simulink model "c6_goto_target"  (R2021b)
settings: Solver=FixedStepDiscrete  StartTime=0.0  StopTime=Inf  FixedStep=sampleTime  RelTol=1e-3  EnableMultiTasking=on
PreLoadFcn:
  | %load emptyMap
InitFcn:
  | sampleTime = 0.05;
  | nMedianSize=3;
  | %load boundaryMap
  | 
  | % Robot parameters
  | wheelRadius = 0.0303;
  | robotRadius = 0.06;   %小车在仿真中显示的圆形的半径大小
  | Trackwidth = 0.0847;  %定义向量场直方图算法中小车的宽度
  | 
  | % Lidar parameters
  | sensorOffset = [0,0];
  | scanAngles = linspace(-pi/3,pi/3,20)';%y = linspace(x1,x2,n) 生成 n 个点。这些点的间距为 (x2-x1)/(n-1)。
  | maxRange = 0.4;
  | 
  | %%%%%%
  | ks=1;
  | 
  | 
  | 
  | 
  | 
  | A=0.5;
  | C=1.5;
  | B=(A+C)/2;
  | 
  | wp1=[A,A; B,A;  C,A; C,B;C,C; B,C; A,C;A,B];
  | bainjie2=[-0.5,-0.5;2.5,-0.5;-0.5,2.5;2.5,2.5;]
  | WAY_P=[wp1;wp1;wp1;wp1];
  | Target=[wp1;bainjie2];
  | 
  | %%%%%%%%%%%%%%%%%%%%%%%%%%%%%%%%%%%%%%%
  | Target_robot_4=[A  A]
  | Target_robot_5=[B  A]
  | Target_robot_6=[C  A]
  | 
  | Target_robot_1=[C  C]
  | Target_robot_2=[B  C]
  | Target_robot_3=[A  C]
  | 
  | 
  | %%%%%%%%%%%%%%%%%%%%%%%%%%%%%%%%%%%%
  | 
  | 
  | init_pose_1=[A    A  pi/2]';
  | init_pose_2=[B    A  pi/2]';
  | init_pose_3=[C    A  pi/2]';
  | init_pose_4=[C    C  -pi/2]';
  | init_pose_5=[B    C  -pi/2]';
  | init_pose_6=[A    C  -pi/2]';
  | 
  | 
  | 
  | 
  | %{
  | %初始位置 交叉
  | 
  | init_pose_1=[C    C    0]';
  | init_pose_2=[B    C    0]';
  | init_pose_3=[A    C  0]';
  | init_pose_4=[A    A  0]';
  | ... (+26 lines)
undefined symbols (not defined in the file or in its folder): Angular, DiscIntNeverNeededParam, Linear
libraries: robotlib x27, dspstat3 x18, robotalgslib x12
(part 2 of 3)

== system c6_goto_target/controller1/Subsystem2/Compute Velocity and Heading for Path following ==
  note: Check If Close To Goal
  CurrentPose : Inport
  Waypoints : Inport  Port=2
  " Extract Goal" : MATLAB Function  TreatAsAtomicUnit=on
  Dot Product : DotProduct  InputSameDT=on  OutDataTypeStr=Inherit: Inherit via internal rule
  GoalRadius : Constant  Value=0.1
  Pure Pursuit : robotalgslib/Pure Pursuit  DesiredLinearVelocity=desired_v  MaxAngularVelocity=desired_w  LookaheadDistance=desired_lookahead  TargetDirPort=on  SimulateUsing=Code generation
  Relational Operator : RelationalOperator  Operator=<=  OutDataTypeStr=boolean  RndMeth=Simplest
  Selector : Selector  InputPortWidth=3  IndexOptions=Index vector (dialog)  Indices=[1 2]  OutputSizes=1
  Sqrt : Sqrt  SaturateOnIntegerOverflow=on
  Subtract : Sum  Inputs=+-
  TargetDir : Outport  VectorParamsAs1DForOutWhenUnconnected=off
  V : Outport  Port=2  VectorParamsAs1DForOutWhenUnconnected=off
  W : Outport  Port=3  VectorParamsAs1DForOutWhenUnconnected=off
  CloseToGoal : Outport  Port=4  VectorParamsAs1DForOutWhenUnconnected=off
  wires:
  Pure Pursuit/3 -> TargetDir/1
  Pure Pursuit/2 -> W/1
  Pure Pursuit/1 -> V/1
  " Extract Goal"/1(Goal) -> Subtract/2
  Waypoints/1 -> " Extract Goal"/1(Waypoints), Pure Pursuit/2
  CurrentPose/1 -> Selector/1, Pure Pursuit/1
  Relational Operator/1 -> CloseToGoal/1
  GoalRadius/1 -> Relational Operator/2
  Selector/1 -> Subtract/1
  Dot Product/1 -> Sqrt/1
  Sqrt/1 -> Relational Operator/1
  Subtract/1 -> Dot Product/1, Dot Product/2

== system c6_goto_target/controller1/Subsystem2/More Info ==

== system c6_goto_target/controller1/Subsystem2/Outputs ==
  dV : Inport
  dW : Inport  Port=2
  V : Inport  Port=3
  W : Inport  Port=4
  CloseToGoal : Inport  Port=5
  Add : Sum
  Add1 : Sum
  Logical Operator : Logic  Operator=NOT  AllPortsSameDT=off  OutDataTypeStr=boolean
  Product : Product
  Product1 : Product
  v : Outport
  w : Outport  Port=2
  wires:
  V/1 -> Add/2
  W/1 -> Add1/2
  dV/1 -> Add/1
  dW/1 -> Add1/1
  CloseToGoal/1 -> Logical Operator/1
  Add/1 -> Product/1
  Add1/1 -> Product1/1
  Product1/1 -> w/1
  Product/1 -> v/1
  Logical Operator/1 -> Product1/2, Product/2

== system c6_goto_target/controller1/Subsystem3/Adjust Velocities to Avoid Obstacles ==
  note: Based on proposed steering direction, evaluate feasible velocities (linear and angular).
      | 				Switch to recovery behavior if no feasible steering direction.
  Ranges : Inport
  Angles : Inport  Port=2
  TargetDir : Inport  Port=3
  V : Inport  Port=4
  W : Inport  Port=5
  If : If  IfExpression=u1 == 1
  Merge : Merge
  Merge1 : Merge
  Path Following : Subsystem  TreatAsAtomicUnit=on
  Recovery : Subsystem  TreatAsAtomicUnit=on
  Relational Operator : RelationalOperator  Operator=isNaN  OutDataTypeStr=boolean  RndMeth=Simplest
  Vector Field Histogram : robotalgslib/Vector Field Histogram  NumAngularSectors=180  DistanceLimits=[ 0.05, 3 ]  HistogramThresholds=[ 3, 8 ]  RobotRadius=0.2  SafetyDistance=0.2  MinTurningRadius=0.2  SimulateUsing=Code generation  TargetDirectionWeight=5  CurrentDirectionWeight=2  PreviousDirectionWeight=2
      settings: SourceProductBaseCode=NV,RO
  dV : Outport  VectorParamsAs1DForOutWhenUnconnected=off
  dW : Outport  Port=2  VectorParamsAs1DForOutWhenUnconnected=off
  wires:
  Merge1/1 -> dW/1
  V/1 -> Recovery/1(LinearVelocity)
  Vector Field Histogram/1 -> Relational Operator/1, Path Following/1(SteeringDirection)
  W/1 -> Recovery/2(AngularVelocity), Path Following/2(AngularVelocity)
  Relational Operator/1 -> If/1
  Angles/1 -> Vector Field Histogram/2
  Merge/1 -> dV/1
  TargetDir/1 -> Vector Field Histogram/3
  Ranges/1 -> Vector Field Histogram/1
  If/1 -> Recovery/Action
  If/2 -> Path Following/Action
  Recovery/2(dW) -> Merge1/1
  Path Following/2(dW) -> Merge1/2
  Recovery/1(dV) -> Merge/1
  Path Following/1(dV) -> Merge/2

== system c6_goto_target/controller1/Subsystem3/Compute Velocity and Heading for Path following ==
  note: Check If Close To Goal
  CurrentPose : Inport
  Waypoints : Inport  Port=2
  " Extract Goal" : MATLAB Function  TreatAsAtomicUnit=on
  Dot Product : DotProduct  InputSameDT=on  OutDataTypeStr=Inherit: Inherit via internal rule
  GoalRadius : Constant  Value=0.1
  Pure Pursuit : robotalgslib/Pure Pursuit  DesiredLinearVelocity=desired_v  MaxAngularVelocity=desired_w  LookaheadDistance=desired_lookahead  TargetDirPort=on  SimulateUsing=Code generation
  Relational Operator : RelationalOperator  Operator=<=  OutDataTypeStr=boolean  RndMeth=Simplest
  Selector : Selector  InputPortWidth=3  IndexOptions=Index vector (dialog)  Indices=[1 2]  OutputSizes=1
  Sqrt : Sqrt  SaturateOnIntegerOverflow=on
  Subtract : Sum  Inputs=+-
  TargetDir : Outport  VectorParamsAs1DForOutWhenUnconnected=off
  V : Outport  Port=2  VectorParamsAs1DForOutWhenUnconnected=off
  W : Outport  Port=3  VectorParamsAs1DForOutWhenUnconnected=off
  CloseToGoal : Outport  Port=4  VectorParamsAs1DForOutWhenUnconnected=off
  wires:
  Pure Pursuit/3 -> TargetDir/1
  Pure Pursuit/2 -> W/1
  Pure Pursuit/1 -> V/1
  " Extract Goal"/1(Goal) -> Subtract/2
  Waypoints/1 -> " Extract Goal"/1(Waypoints), Pure Pursuit/2
  CurrentPose/1 -> Selector/1, Pure Pursuit/1
  Relational Operator/1 -> CloseToGoal/1
  GoalRadius/1 -> Relational Operator/2
  Selector/1 -> Subtract/1
  Dot Product/1 -> Sqrt/1
  Sqrt/1 -> Relational Operator/1
  Subtract/1 -> Dot Product/1, Dot Product/2

== system c6_goto_target/controller1/Subsystem3/More Info ==

== system c6_goto_target/controller1/Subsystem3/Outputs ==
  dV : Inport
  dW : Inport  Port=2
  V : Inport  Port=3
  W : Inport  Port=4
  CloseToGoal : Inport  Port=5
  Add : Sum
  Add1 : Sum
  Logical Operator : Logic  Operator=NOT  AllPortsSameDT=off  OutDataTypeStr=boolean
  Product : Product
  Product1 : Product
  v : Outport
  w : Outport  Port=2
  wires:
  V/1 -> Add/2
  W/1 -> Add1/2
  dV/1 -> Add/1
  dW/1 -> Add1/1
  CloseToGoal/1 -> Logical Operator/1
  Add/1 -> Product/1
  Add1/1 -> Product1/1
  Product1/1 -> w/1
  Product/1 -> v/1
  Logical Operator/1 -> Product1/2, Product/2

== system c6_goto_target/controller1/Subsystem4/Adjust Velocities to Avoid Obstacles ==
  note: Based on proposed steering direction, evaluate feasible velocities (linear and angular).
      | 				Switch to recovery behavior if no feasible steering direction.
  Ranges : Inport
  Angles : Inport  Port=2
  TargetDir : Inport  Port=3
  V : Inport  Port=4
  W : Inport  Port=5
  If : If  IfExpression=u1 == 1
  Merge : Merge
  Merge1 : Merge
  Path Following : Subsystem  TreatAsAtomicUnit=on
  Recovery : Subsystem  TreatAsAtomicUnit=on
  Relational Operator : RelationalOperator  Operator=isNaN  OutDataTypeStr=boolean  RndMeth=Simplest
  Vector Field Histogram : robotalgslib/Vector Field Histogram  NumAngularSectors=180  DistanceLimits=[ 0.05, 3 ]  HistogramThresholds=[ 3, 8 ]  RobotRadius=0.2  SafetyDistance=0.2  MinTurningRadius=0.2  SimulateUsing=Code generation  TargetDirectionWeight=5  CurrentDirectionWeight=2  PreviousDirectionWeight=2
      settings: SourceProductBaseCode=NV,RO
  dV : Outport  VectorParamsAs1DForOutWhenUnconnected=off
  dW : Outport  Port=2  VectorParamsAs1DForOutWhenUnconnected=off
  wires:
  Merge1/1 -> dW/1
  V/1 -> Recovery/1(LinearVelocity)
  Vector Field Histogram/1 -> Relational Operator/1, Path Following/1(SteeringDirection)
  W/1 -> Recovery/2(AngularVelocity), Path Following/2(AngularVelocity)
  Relational Operator/1 -> If/1
  Angles/1 -> Vector Field Histogram/2
  Merge/1 -> dV/1
  TargetDir/1 -> Vector Field Histogram/3
  Ranges/1 -> Vector Field Histogram/1
  If/1 -> Recovery/Action
  If/2 -> Path Following/Action
  Recovery/2(dW) -> Merge1/1
  Path Following/2(dW) -> Merge1/2
  Recovery/1(dV) -> Merge/1
  Path Following/1(dV) -> Merge/2

== system c6_goto_target/controller1/Subsystem4/Compute Velocity and Heading for Path following ==
  note: Check If Close To Goal
  CurrentPose : Inport
  Waypoints : Inport  Port=2
  " Extract Goal" : MATLAB Function  TreatAsAtomicUnit=on
  Dot Product : DotProduct  InputSameDT=on  OutDataTypeStr=Inherit: Inherit via internal rule
  GoalRadius : Constant  Value=0.1
  Pure Pursuit : robotalgslib/Pure Pursuit  DesiredLinearVelocity=desired_v  MaxAngularVelocity=desired_w  LookaheadDistance=desired_lookahead  TargetDirPort=on  SimulateUsing=Code generation
  Relational Operator : RelationalOperator  Operator=<=  OutDataTypeStr=boolean  RndMeth=Simplest
  Selector : Selector  InputPortWidth=3  IndexOptions=Index vector (dialog)  Indices=[1 2]  OutputSizes=1
  Sqrt : Sqrt  SaturateOnIntegerOverflow=on
  Subtract : Sum  Inputs=+-
  TargetDir : Outport  VectorParamsAs1DForOutWhenUnconnected=off
  V : Outport  Port=2  VectorParamsAs1DForOutWhenUnconnected=off
  W : Outport  Port=3  VectorParamsAs1DForOutWhenUnconnected=off
  CloseToGoal : Outport  Port=4  VectorParamsAs1DForOutWhenUnconnected=off
  wires:
  Pure Pursuit/3 -> TargetDir/1
  Pure Pursuit/2 -> W/1
  Pure Pursuit/1 -> V/1
  " Extract Goal"/1(Goal) -> Subtract/2
  Waypoints/1 -> " Extract Goal"/1(Waypoints), Pure Pursuit/2
  CurrentPose/1 -> Selector/1, Pure Pursuit/1
  Relational Operator/1 -> CloseToGoal/1
  GoalRadius/1 -> Relational Operator/2
  Selector/1 -> Subtract/1
  Dot Product/1 -> Sqrt/1
  Sqrt/1 -> Relational Operator/1
  Subtract/1 -> Dot Product/1, Dot Product/2

== system c6_goto_target/controller1/Subsystem4/More Info ==

== system c6_goto_target/controller1/Subsystem4/Outputs ==
  dV : Inport
  dW : Inport  Port=2
  V : Inport  Port=3
  W : Inport  Port=4
  CloseToGoal : Inport  Port=5
  Add : Sum
  Add1 : Sum
  Logical Operator : Logic  Operator=NOT  AllPortsSameDT=off  OutDataTypeStr=boolean
  Product : Product
  Product1 : Product
  v : Outport
  w : Outport  Port=2
  wires:
  V/1 -> Add/2
  W/1 -> Add1/2
  dV/1 -> Add/1
  dW/1 -> Add1/1
  CloseToGoal/1 -> Logical Operator/1
  Add/1 -> Product/1
  Add1/1 -> Product1/1
  Product1/1 -> w/1
  Product/1 -> v/1
  Logical Operator/1 -> Product1/2, Product/2

== system c6_goto_target/controller1/Subsystem5/Adjust Velocities to Avoid Obstacles ==
  note: Based on proposed steering direction, evaluate feasible velocities (linear and angular).
      | 				Switch to recovery behavior if no feasible steering direction.
  Ranges : Inport
  Angles : Inport  Port=2
  TargetDir : Inport  Port=3
  V : Inport  Port=4
  W : Inport  Port=5
  If : If  IfExpression=u1 == 1
  Merge : Merge
  Merge1 : Merge
  Path Following : Subsystem  TreatAsAtomicUnit=on
  Recovery : Subsystem  TreatAsAtomicUnit=on
  Relational Operator : RelationalOperator  Operator=isNaN  OutDataTypeStr=boolean  RndMeth=Simplest
  Vector Field Histogram : robotalgslib/Vector Field Histogram  NumAngularSectors=180  DistanceLimits=[ 0.05, 3 ]  HistogramThresholds=[ 3, 8 ]  RobotRadius=0.2  SafetyDistance=0.2  MinTurningRadius=0.2  SimulateUsing=Code generation  TargetDirectionWeight=5  CurrentDirectionWeight=2  PreviousDirectionWeight=2
      settings: SourceProductBaseCode=NV,RO
  dV : Outport  VectorParamsAs1DForOutWhenUnconnected=off
  dW : Outport  Port=2  VectorParamsAs1DForOutWhenUnconnected=off
  wires:
  Merge1/1 -> dW/1
  V/1 -> Recovery/1(LinearVelocity)
  Vector Field Histogram/1 -> Relational Operator/1, Path Following/1(SteeringDirection)
  W/1 -> Recovery/2(AngularVelocity), Path Following/2(AngularVelocity)
  Relational Operator/1 -> If/1
  Angles/1 -> Vector Field Histogram/2
  Merge/1 -> dV/1
  TargetDir/1 -> Vector Field Histogram/3
  Ranges/1 -> Vector Field Histogram/1
  If/1 -> Recovery/Action
  If/2 -> Path Following/Action
  Recovery/2(dW) -> Merge1/1
  Path Following/2(dW) -> Merge1/2
  Recovery/1(dV) -> Merge/1
  Path Following/1(dV) -> Merge/2

== system c6_goto_target/controller1/Subsystem5/Compute Velocity and Heading for Path following ==
  note: Check If Close To Goal
  CurrentPose : Inport
  Waypoints : Inport  Port=2
  " Extract Goal" : MATLAB Function  TreatAsAtomicUnit=on
  Dot Product : DotProduct  InputSameDT=on  OutDataTypeStr=Inherit: Inherit via internal rule
  GoalRadius : Constant  Value=0.1
  Pure Pursuit : robotalgslib/Pure Pursuit  DesiredLinearVelocity=desired_v  MaxAngularVelocity=desired_w  LookaheadDistance=desired_lookahead  TargetDirPort=on  SimulateUsing=Code generation
  Relational Operator : RelationalOperator  Operator=<=  OutDataTypeStr=boolean  RndMeth=Simplest
  Selector : Selector  InputPortWidth=3  IndexOptions=Index vector (dialog)  Indices=[1 2]  OutputSizes=1
  Sqrt : Sqrt  SaturateOnIntegerOverflow=on
  Subtract : Sum  Inputs=+-
  TargetDir : Outport  VectorParamsAs1DForOutWhenUnconnected=off
  V : Outport  Port=2  VectorParamsAs1DForOutWhenUnconnected=off
  W : Outport  Port=3  VectorParamsAs1DForOutWhenUnconnected=off
  CloseToGoal : Outport  Port=4  VectorParamsAs1DForOutWhenUnconnected=off
  wires:
  Pure Pursuit/3 -> TargetDir/1
  Pure Pursuit/2 -> W/1
  Pure Pursuit/1 -> V/1
  " Extract Goal"/1(Goal) -> Subtract/2
  Waypoints/1 -> " Extract Goal"/1(Waypoints), Pure Pursuit/2
  CurrentPose/1 -> Selector/1, Pure Pursuit/1
  Relational Operator/1 -> CloseToGoal/1
  GoalRadius/1 -> Relational Operator/2
  Selector/1 -> Subtract/1
  Dot Product/1 -> Sqrt/1
  Sqrt/1 -> Relational Operator/1
  Subtract/1 -> Dot Product/1, Dot Product/2

== system c6_goto_target/controller1/Subsystem5/More Info ==

== system c6_goto_target/controller1/Subsystem5/Outputs ==
  dV : Inport
  dW : Inport  Port=2
  V : Inport  Port=3
  W : Inport  Port=4
  CloseToGoal : Inport  Port=5
  Add : Sum
  Add1 : Sum
  Logical Operator : Logic  Operator=NOT  AllPortsSameDT=off  OutDataTypeStr=boolean
  Product : Product
  Product1 : Product
  v : Outport
  w : Outport  Port=2
  wires:
  V/1 -> Add/2
  W/1 -> Add1/2
  dV/1 -> Add/1
  dW/1 -> Add1/1
  CloseToGoal/1 -> Logical Operator/1
  Add/1 -> Product/1
  Add1/1 -> Product1/1
  Product1/1 -> w/1
  Product/1 -> v/1
  Logical Operator/1 -> Product1/2, Product/2

== system c6_goto_target/controller1/Subsystem6/Adjust Velocities to Avoid Obstacles ==
  note: Based on proposed steering direction, evaluate feasible velocities (linear and angular).
      | 				Switch to recovery behavior if no feasible steering direction.
  Ranges : Inport
  Angles : Inport  Port=2
  TargetDir : Inport  Port=3
  V : Inport  Port=4
  W : Inport  Port=5
  If : If  IfExpression=u1 == 1
  Merge : Merge
  Merge1 : Merge
  Path Following : Subsystem  TreatAsAtomicUnit=on
  Recovery : Subsystem  TreatAsAtomicUnit=on
  Relational Operator : RelationalOperator  Operator=isNaN  OutDataTypeStr=boolean  RndMeth=Simplest
  Vector Field Histogram : robotalgslib/Vector Field Histogram  NumAngularSectors=180  DistanceLimits=[ 0.05, 3 ]  HistogramThresholds=[ 3, 8 ]  RobotRadius=0.2  SafetyDistance=0.2  MinTurningRadius=0.2  SimulateUsing=Code generation  TargetDirectionWeight=5  CurrentDirectionWeight=2  PreviousDirectionWeight=2
      settings: SourceProductBaseCode=NV,RO
  dV : Outport  VectorParamsAs1DForOutWhenUnconnected=off
  dW : Outport  Port=2  VectorParamsAs1DForOutWhenUnconnected=off
  wires:
  Merge1/1 -> dW/1
  V/1 -> Recovery/1(LinearVelocity)
  Vector Field Histogram/1 -> Relational Operator/1, Path Following/1(SteeringDirection)
  W/1 -> Recovery/2(AngularVelocity), Path Following/2(AngularVelocity)
  Relational Operator/1 -> If/1
  Angles/1 -> Vector Field Histogram/2
  Merge/1 -> dV/1
  TargetDir/1 -> Vector Field Histogram/3
  Ranges/1 -> Vector Field Histogram/1
  If/1 -> Recovery/Action
  If/2 -> Path Following/Action
  Recovery/2(dW) -> Merge1/1
  Path Following/2(dW) -> Merge1/2
  Recovery/1(dV) -> Merge/1
  Path Following/1(dV) -> Merge/2

== system c6_goto_target/controller1/Subsystem6/Compute Velocity and Heading for Path following ==
  note: Check If Close To Goal
  CurrentPose : Inport
  Waypoints : Inport  Port=2
  " Extract Goal" : MATLAB Function  TreatAsAtomicUnit=on
  Dot Product : DotProduct  InputSameDT=on  OutDataTypeStr=Inherit: Inherit via internal rule
  GoalRadius : Constant  Value=0.1
  Pure Pursuit : robotalgslib/Pure Pursuit  DesiredLinearVelocity=desired_v  MaxAngularVelocity=desired_w  LookaheadDistance=desired_lookahead  TargetDirPort=on  SimulateUsing=Code generation
  Relational Operator : RelationalOperator  Operator=<=  OutDataTypeStr=boolean  RndMeth=Simplest
  Selector : Selector  InputPortWidth=3  IndexOptions=Index vector (dialog)  Indices=[1 2]  OutputSizes=1
  Sqrt : Sqrt  SaturateOnIntegerOverflow=on
  Subtract : Sum  Inputs=+-
  TargetDir : Outport  VectorParamsAs1DForOutWhenUnconnected=off
  V : Outport  Port=2  VectorParamsAs1DForOutWhenUnconnected=off
  W : Outport  Port=3  VectorParamsAs1DForOutWhenUnconnected=off
  CloseToGoal : Outport  Port=4  VectorParamsAs1DForOutWhenUnconnected=off
  wires:
  Pure Pursuit/3 -> TargetDir/1
  Pure Pursuit/2 -> W/1
  Pure Pursuit/1 -> V/1
  " Extract Goal"/1(Goal) -> Subtract/2
  Waypoints/1 -> " Extract Goal"/1(Waypoints), Pure Pursuit/2
  CurrentPose/1 -> Selector/1, Pure Pursuit/1
  Relational Operator/1 -> CloseToGoal/1
  GoalRadius/1 -> Relational Operator/2
  Selector/1 -> Subtract/1
  Dot Product/1 -> Sqrt/1
  Sqrt/1 -> Relational Operator/1
  Subtract/1 -> Dot Product/1, Dot Product/2

== system c6_goto_target/controller1/Subsystem6/More Info ==

== system c6_goto_target/controller1/Subsystem6/Outputs ==
  dV : Inport
  dW : Inport  Port=2
  V : Inport  Port=3
  W : Inport  Port=4
  CloseToGoal : Inport  Port=5
  Add : Sum
  Add1 : Sum
  Logical Operator : Logic  Operator=NOT  AllPortsSameDT=off  OutDataTypeStr=boolean
  Product : Product
  Product1 : Product
  v : Outport
  w : Outport  Port=2
  wires:
  V/1 -> Add/2
  W/1 -> Add1/2
  dV/1 -> Add/1
  dW/1 -> Add1/1
  CloseToGoal/1 -> Logical Operator/1
  Add/1 -> Product/1
  Add1/1 -> Product1/1
  Product1/1 -> w/1
  Product/1 -> v/1
  Logical Operator/1 -> Product1/2, Product/2

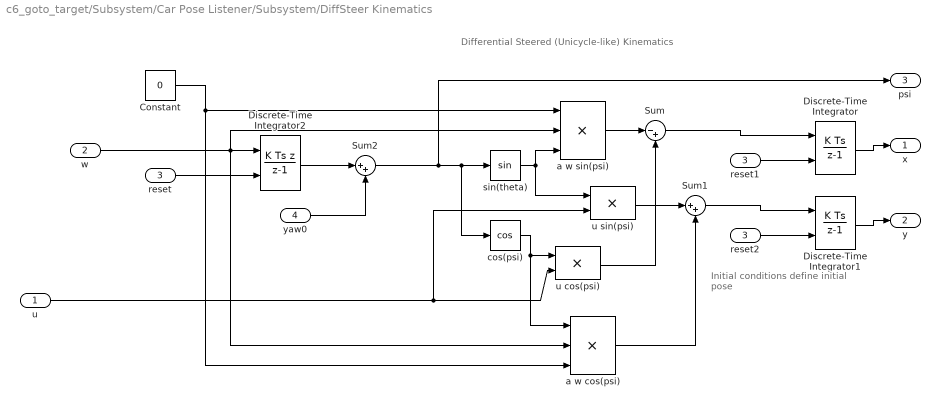
== system c6_goto_target/Subsystem/Car Pose Listener/Subsystem/DiffSteer Kinematics ==
  note: Initial conditions define
      | initial pose
  note: Differential Steered (Unicycle-like) Kinematics
  u : Inport
  w : Inport  Port=2
  reset : Inport  Port=3
  yaw0 : Inport  Port=4
  Constant : Constant  Value=0
  Discrete-Time Integrator : DiscreteIntegrator  ExternalReset=falling  SampleTime=-1  ICPrevOutput=DiscIntNeverNeededParam  ICPrevScaledInput=DiscIntNeverNeededParam
  Discrete-Time Integrator1 : DiscreteIntegrator  ExternalReset=falling  SampleTime=-1  ICPrevOutput=DiscIntNeverNeededParam  ICPrevScaledInput=DiscIntNeverNeededParam
  Discrete-Time Integrator2 : DiscreteIntegrator  IntegratorMethod=Integration: Backward Euler  ExternalReset=falling  SampleTime=-1  ICPrevOutput=DiscIntNeverNeededParam  ICPrevScaledInput=DiscIntNeverNeededParam
  Sum : Sum  Inputs=|-+  SaturateOnIntegerOverflow=on
  Sum1 : Sum  Inputs=|++  SaturateOnIntegerOverflow=on
  Sum2 : Sum  Inputs=|++
  a w cos(psi) : Product  Inputs=3  SaturateOnIntegerOverflow=on  OutDataTypeStr=Inherit: Same as first input
  a w sin(psi) : Product  Inputs=3  SaturateOnIntegerOverflow=on  OutDataTypeStr=Inherit: Same as first input
  cos(psi) : Trigonometry  Operator=cos
  reset1 : InportShadow  Port=3
  reset2 : InportShadow  Port=3
  sin(theta) : Trigonometry
  u cos(psi) : Product  SaturateOnIntegerOverflow=on  OutDataTypeStr=Inherit: Same as first input
  u sin(psi) : Product  SaturateOnIntegerOverflow=on  OutDataTypeStr=Inherit: Same as first input
  x : Outport
  y : Outport  Port=2
  psi : Outport  Port=3
  wires:
  yaw0/1 -> Sum2/2
  reset2/1 -> Discrete-Time Integrator1/2
  reset1/1 -> Discrete-Time Integrator/2
  reset/1 -> Discrete-Time Integrator2/2
  u sin(psi)/1 -> Sum1/1
  cos(psi)/1 -> u cos(psi)/1, a w cos(psi)/1
  w/1 -> a w cos(psi)/2, a w sin(psi)/2, Discrete-Time Integrator2/1
  Constant/1 -> a w sin(psi)/1, a w cos(psi)/3
  Discrete-Time Integrator/1 -> x/1
  Sum/1 -> Discrete-Time Integrator/1
  sin(theta)/1 -> a w sin(psi)/3, u sin(psi)/1
  a w cos(psi)/1 -> Sum1/2
  Sum2/1 -> psi/1, sin(theta)/1, cos(psi)/1
  u cos(psi)/1 -> Sum/2
  u/1 -> u sin(psi)/2, u cos(psi)/2
  a w sin(psi)/1 -> Sum/1
  Sum1/1 -> Discrete-Time Integrator1/1
  Discrete-Time Integrator1/1 -> y/1
  Discrete-Time Integrator2/1 -> Sum2/1

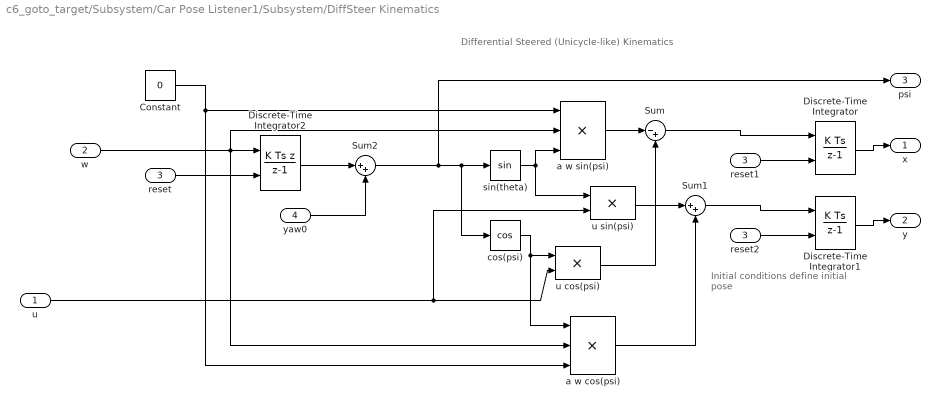
== system c6_goto_target/Subsystem/Car Pose Listener1/Subsystem/DiffSteer Kinematics ==
  note: Initial conditions define
      | initial pose
  note: Differential Steered (Unicycle-like) Kinematics
  u : Inport
  w : Inport  Port=2
  reset : Inport  Port=3
  yaw0 : Inport  Port=4
  Constant : Constant  Value=0
  Discrete-Time Integrator : DiscreteIntegrator  ExternalReset=falling  SampleTime=-1  ICPrevOutput=DiscIntNeverNeededParam  ICPrevScaledInput=DiscIntNeverNeededParam
  Discrete-Time Integrator1 : DiscreteIntegrator  ExternalReset=falling  SampleTime=-1  ICPrevOutput=DiscIntNeverNeededParam  ICPrevScaledInput=DiscIntNeverNeededParam
  Discrete-Time Integrator2 : DiscreteIntegrator  IntegratorMethod=Integration: Backward Euler  ExternalReset=falling  SampleTime=-1  ICPrevOutput=DiscIntNeverNeededParam  ICPrevScaledInput=DiscIntNeverNeededParam
  Sum : Sum  Inputs=|-+  SaturateOnIntegerOverflow=on
  Sum1 : Sum  Inputs=|++  SaturateOnIntegerOverflow=on
  Sum2 : Sum  Inputs=|++
  a w cos(psi) : Product  Inputs=3  SaturateOnIntegerOverflow=on  OutDataTypeStr=Inherit: Same as first input
  a w sin(psi) : Product  Inputs=3  SaturateOnIntegerOverflow=on  OutDataTypeStr=Inherit: Same as first input
  cos(psi) : Trigonometry  Operator=cos
  reset1 : InportShadow  Port=3
  reset2 : InportShadow  Port=3
  sin(theta) : Trigonometry
  u cos(psi) : Product  SaturateOnIntegerOverflow=on  OutDataTypeStr=Inherit: Same as first input
  u sin(psi) : Product  SaturateOnIntegerOverflow=on  OutDataTypeStr=Inherit: Same as first input
  x : Outport
  y : Outport  Port=2
  psi : Outport  Port=3
  wires:
  yaw0/1 -> Sum2/2
  reset2/1 -> Discrete-Time Integrator1/2
  reset1/1 -> Discrete-Time Integrator/2
  reset/1 -> Discrete-Time Integrator2/2
  u sin(psi)/1 -> Sum1/1
  cos(psi)/1 -> u cos(psi)/1, a w cos(psi)/1
  w/1 -> a w cos(psi)/2, a w sin(psi)/2, Discrete-Time Integrator2/1
  Constant/1 -> a w sin(psi)/1, a w cos(psi)/3
  Discrete-Time Integrator/1 -> x/1
  Sum/1 -> Discrete-Time Integrator/1
  sin(theta)/1 -> a w sin(psi)/3, u sin(psi)/1
  a w cos(psi)/1 -> Sum1/2
  Sum2/1 -> psi/1, sin(theta)/1, cos(psi)/1
  u cos(psi)/1 -> Sum/2
  u/1 -> u sin(psi)/2, u cos(psi)/2
  a w sin(psi)/1 -> Sum/1
  Sum1/1 -> Discrete-Time Integrator1/1
  Discrete-Time Integrator1/1 -> y/1
  Discrete-Time Integrator2/1 -> Sum2/1

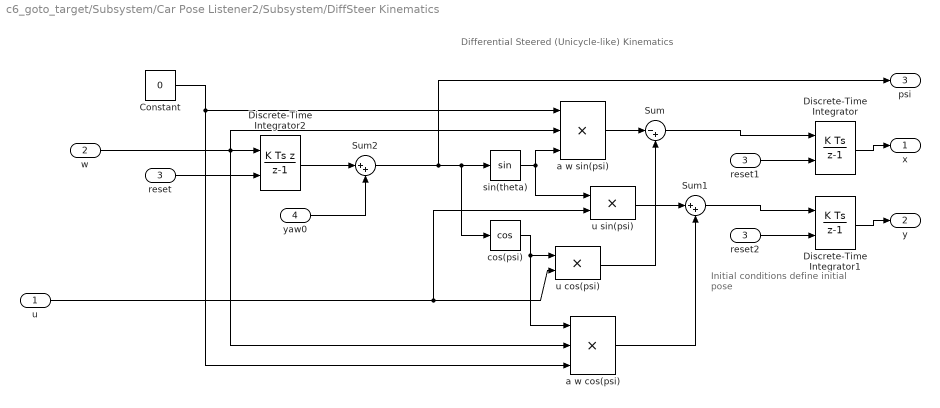
== system c6_goto_target/Subsystem/Car Pose Listener2/Subsystem/DiffSteer Kinematics ==
  note: Initial conditions define
      | initial pose
  note: Differential Steered (Unicycle-like) Kinematics
  u : Inport
  w : Inport  Port=2
  reset : Inport  Port=3
  yaw0 : Inport  Port=4
  Constant : Constant  Value=0
  Discrete-Time Integrator : DiscreteIntegrator  ExternalReset=falling  SampleTime=-1  ICPrevOutput=DiscIntNeverNeededParam  ICPrevScaledInput=DiscIntNeverNeededParam
  Discrete-Time Integrator1 : DiscreteIntegrator  ExternalReset=falling  SampleTime=-1  ICPrevOutput=DiscIntNeverNeededParam  ICPrevScaledInput=DiscIntNeverNeededParam
  Discrete-Time Integrator2 : DiscreteIntegrator  IntegratorMethod=Integration: Backward Euler  ExternalReset=falling  SampleTime=-1  ICPrevOutput=DiscIntNeverNeededParam  ICPrevScaledInput=DiscIntNeverNeededParam
  Sum : Sum  Inputs=|-+  SaturateOnIntegerOverflow=on
  Sum1 : Sum  Inputs=|++  SaturateOnIntegerOverflow=on
  Sum2 : Sum  Inputs=|++
  a w cos(psi) : Product  Inputs=3  SaturateOnIntegerOverflow=on  OutDataTypeStr=Inherit: Same as first input
  a w sin(psi) : Product  Inputs=3  SaturateOnIntegerOverflow=on  OutDataTypeStr=Inherit: Same as first input
  cos(psi) : Trigonometry  Operator=cos
  reset1 : InportShadow  Port=3
  reset2 : InportShadow  Port=3
  sin(theta) : Trigonometry
  u cos(psi) : Product  SaturateOnIntegerOverflow=on  OutDataTypeStr=Inherit: Same as first input
  u sin(psi) : Product  SaturateOnIntegerOverflow=on  OutDataTypeStr=Inherit: Same as first input
  x : Outport
  y : Outport  Port=2
  psi : Outport  Port=3
  wires:
  yaw0/1 -> Sum2/2
  reset2/1 -> Discrete-Time Integrator1/2
  reset1/1 -> Discrete-Time Integrator/2
  reset/1 -> Discrete-Time Integrator2/2
  u sin(psi)/1 -> Sum1/1
  cos(psi)/1 -> u cos(psi)/1, a w cos(psi)/1
  w/1 -> a w cos(psi)/2, a w sin(psi)/2, Discrete-Time Integrator2/1
  Constant/1 -> a w sin(psi)/1, a w cos(psi)/3
  Discrete-Time Integrator/1 -> x/1
  Sum/1 -> Discrete-Time Integrator/1
  sin(theta)/1 -> a w sin(psi)/3, u sin(psi)/1
  a w cos(psi)/1 -> Sum1/2
  Sum2/1 -> psi/1, sin(theta)/1, cos(psi)/1
  u cos(psi)/1 -> Sum/2
  u/1 -> u sin(psi)/2, u cos(psi)/2
  a w sin(psi)/1 -> Sum/1
  Sum1/1 -> Discrete-Time Integrator1/1
  Discrete-Time Integrator1/1 -> y/1
  Discrete-Time Integrator2/1 -> Sum2/1

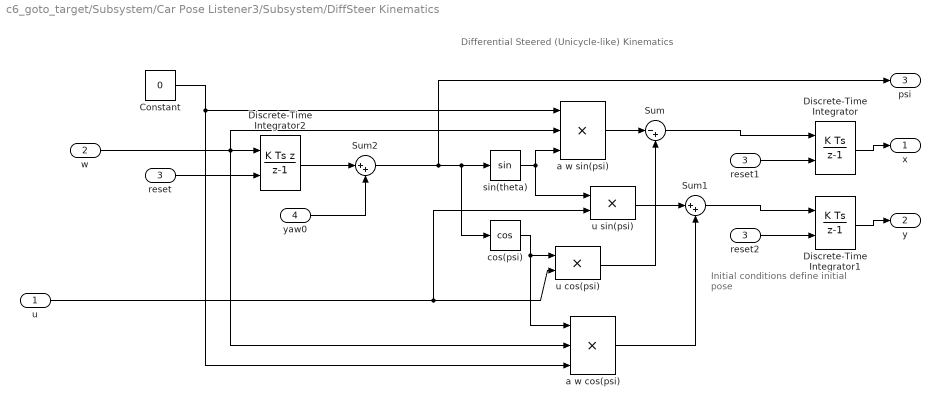
== system c6_goto_target/Subsystem/Car Pose Listener3/Subsystem/DiffSteer Kinematics ==
  note: Initial conditions define
      | initial pose
  note: Differential Steered (Unicycle-like) Kinematics
  u : Inport
  w : Inport  Port=2
  reset : Inport  Port=3
  yaw0 : Inport  Port=4
  Constant : Constant  Value=0
  Discrete-Time Integrator : DiscreteIntegrator  ExternalReset=falling  SampleTime=-1  ICPrevOutput=DiscIntNeverNeededParam  ICPrevScaledInput=DiscIntNeverNeededParam
  Discrete-Time Integrator1 : DiscreteIntegrator  ExternalReset=falling  SampleTime=-1  ICPrevOutput=DiscIntNeverNeededParam  ICPrevScaledInput=DiscIntNeverNeededParam
  Discrete-Time Integrator2 : DiscreteIntegrator  IntegratorMethod=Integration: Backward Euler  ExternalReset=falling  SampleTime=-1  ICPrevOutput=DiscIntNeverNeededParam  ICPrevScaledInput=DiscIntNeverNeededParam
  Sum : Sum  Inputs=|-+  SaturateOnIntegerOverflow=on
  Sum1 : Sum  Inputs=|++  SaturateOnIntegerOverflow=on
  Sum2 : Sum  Inputs=|++
  a w cos(psi) : Product  Inputs=3  SaturateOnIntegerOverflow=on  OutDataTypeStr=Inherit: Same as first input
  a w sin(psi) : Product  Inputs=3  SaturateOnIntegerOverflow=on  OutDataTypeStr=Inherit: Same as first input
  cos(psi) : Trigonometry  Operator=cos
  reset1 : InportShadow  Port=3
  reset2 : InportShadow  Port=3
  sin(theta) : Trigonometry
  u cos(psi) : Product  SaturateOnIntegerOverflow=on  OutDataTypeStr=Inherit: Same as first input
  u sin(psi) : Product  SaturateOnIntegerOverflow=on  OutDataTypeStr=Inherit: Same as first input
  x : Outport
  y : Outport  Port=2
  psi : Outport  Port=3
  wires:
  yaw0/1 -> Sum2/2
  reset2/1 -> Discrete-Time Integrator1/2
  reset1/1 -> Discrete-Time Integrator/2
  reset/1 -> Discrete-Time Integrator2/2
  u sin(psi)/1 -> Sum1/1
  cos(psi)/1 -> u cos(psi)/1, a w cos(psi)/1
  w/1 -> a w cos(psi)/2, a w sin(psi)/2, Discrete-Time Integrator2/1
  Constant/1 -> a w sin(psi)/1, a w cos(psi)/3
  Discrete-Time Integrator/1 -> x/1
  Sum/1 -> Discrete-Time Integrator/1
  sin(theta)/1 -> a w sin(psi)/3, u sin(psi)/1
  a w cos(psi)/1 -> Sum1/2
  Sum2/1 -> psi/1, sin(theta)/1, cos(psi)/1
  u cos(psi)/1 -> Sum/2
  u/1 -> u sin(psi)/2, u cos(psi)/2
  a w sin(psi)/1 -> Sum/1
  Sum1/1 -> Discrete-Time Integrator1/1
  Discrete-Time Integrator1/1 -> y/1
  Discrete-Time Integrator2/1 -> Sum2/1

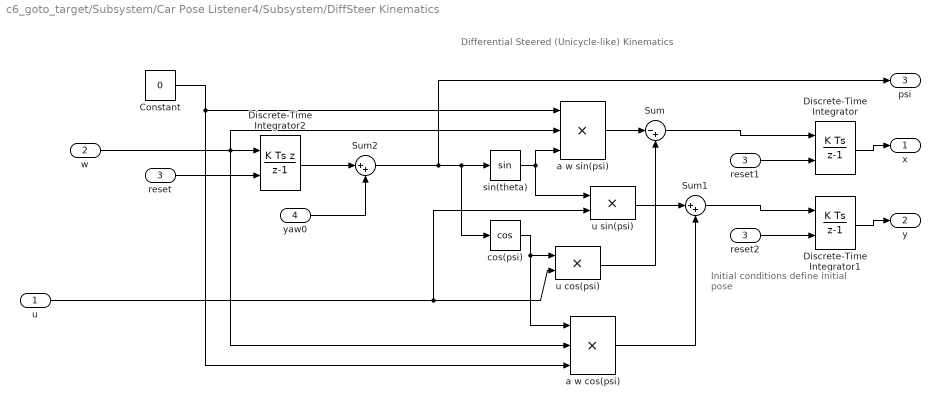
== system c6_goto_target/Subsystem/Car Pose Listener4/Subsystem/DiffSteer Kinematics ==
  note: Initial conditions define
      | initial pose
  note: Differential Steered (Unicycle-like) Kinematics
  u : Inport
  w : Inport  Port=2
  reset : Inport  Port=3
  yaw0 : Inport  Port=4
  Constant : Constant  Value=0
  Discrete-Time Integrator : DiscreteIntegrator  ExternalReset=falling  SampleTime=-1  ICPrevOutput=DiscIntNeverNeededParam  ICPrevScaledInput=DiscIntNeverNeededParam
  Discrete-Time Integrator1 : DiscreteIntegrator  ExternalReset=falling  SampleTime=-1  ICPrevOutput=DiscIntNeverNeededParam  ICPrevScaledInput=DiscIntNeverNeededParam
  Discrete-Time Integrator2 : DiscreteIntegrator  IntegratorMethod=Integration: Backward Euler  ExternalReset=falling  SampleTime=-1  ICPrevOutput=DiscIntNeverNeededParam  ICPrevScaledInput=DiscIntNeverNeededParam
  Sum : Sum  Inputs=|-+  SaturateOnIntegerOverflow=on
  Sum1 : Sum  Inputs=|++  SaturateOnIntegerOverflow=on
  Sum2 : Sum  Inputs=|++
  a w cos(psi) : Product  Inputs=3  SaturateOnIntegerOverflow=on  OutDataTypeStr=Inherit: Same as first input
  a w sin(psi) : Product  Inputs=3  SaturateOnIntegerOverflow=on  OutDataTypeStr=Inherit: Same as first input
  cos(psi) : Trigonometry  Operator=cos
  reset1 : InportShadow  Port=3
  reset2 : InportShadow  Port=3
  sin(theta) : Trigonometry
  u cos(psi) : Product  SaturateOnIntegerOverflow=on  OutDataTypeStr=Inherit: Same as first input
  u sin(psi) : Product  SaturateOnIntegerOverflow=on  OutDataTypeStr=Inherit: Same as first input
  x : Outport
  y : Outport  Port=2
  psi : Outport  Port=3
  wires:
  yaw0/1 -> Sum2/2
  reset2/1 -> Discrete-Time Integrator1/2
  reset1/1 -> Discrete-Time Integrator/2
  reset/1 -> Discrete-Time Integrator2/2
  u sin(psi)/1 -> Sum1/1
  cos(psi)/1 -> u cos(psi)/1, a w cos(psi)/1
  w/1 -> a w cos(psi)/2, a w sin(psi)/2, Discrete-Time Integrator2/1
  Constant/1 -> a w sin(psi)/1, a w cos(psi)/3
  Discrete-Time Integrator/1 -> x/1
  Sum/1 -> Discrete-Time Integrator/1
  sin(theta)/1 -> a w sin(psi)/3, u sin(psi)/1
  a w cos(psi)/1 -> Sum1/2
  Sum2/1 -> psi/1, sin(theta)/1, cos(psi)/1
  u cos(psi)/1 -> Sum/2
  u/1 -> u sin(psi)/2, u cos(psi)/2
  a w sin(psi)/1 -> Sum/1
  Sum1/1 -> Discrete-Time Integrator1/1
  Discrete-Time Integrator1/1 -> y/1
  Discrete-Time Integrator2/1 -> Sum2/1

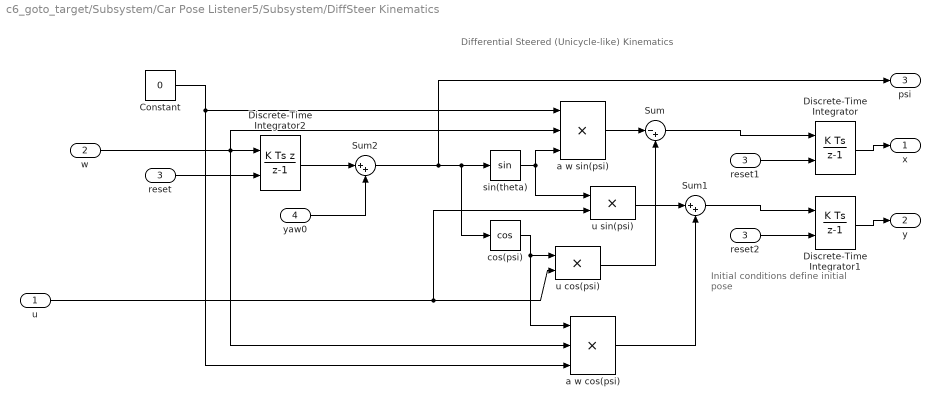
== system c6_goto_target/Subsystem/Car Pose Listener5/Subsystem/DiffSteer Kinematics ==
  note: Initial conditions define
      | initial pose
  note: Differential Steered (Unicycle-like) Kinematics
  u : Inport
  w : Inport  Port=2
  reset : Inport  Port=3
  yaw0 : Inport  Port=4
  Constant : Constant  Value=0
  Discrete-Time Integrator : DiscreteIntegrator  ExternalReset=falling  SampleTime=-1  ICPrevOutput=DiscIntNeverNeededParam  ICPrevScaledInput=DiscIntNeverNeededParam
  Discrete-Time Integrator1 : DiscreteIntegrator  ExternalReset=falling  SampleTime=-1  ICPrevOutput=DiscIntNeverNeededParam  ICPrevScaledInput=DiscIntNeverNeededParam
  Discrete-Time Integrator2 : DiscreteIntegrator  IntegratorMethod=Integration: Backward Euler  ExternalReset=falling  SampleTime=-1  ICPrevOutput=DiscIntNeverNeededParam  ICPrevScaledInput=DiscIntNeverNeededParam
  Sum : Sum  Inputs=|-+  SaturateOnIntegerOverflow=on
  Sum1 : Sum  Inputs=|++  SaturateOnIntegerOverflow=on
  Sum2 : Sum  Inputs=|++
  a w cos(psi) : Product  Inputs=3  SaturateOnIntegerOverflow=on  OutDataTypeStr=Inherit: Same as first input
  a w sin(psi) : Product  Inputs=3  SaturateOnIntegerOverflow=on  OutDataTypeStr=Inherit: Same as first input
  cos(psi) : Trigonometry  Operator=cos
  reset1 : InportShadow  Port=3
  reset2 : InportShadow  Port=3
  sin(theta) : Trigonometry
  u cos(psi) : Product  SaturateOnIntegerOverflow=on  OutDataTypeStr=Inherit: Same as first input
  u sin(psi) : Product  SaturateOnIntegerOverflow=on  OutDataTypeStr=Inherit: Same as first input
  x : Outport
  y : Outport  Port=2
  psi : Outport  Port=3
  wires:
  yaw0/1 -> Sum2/2
  reset2/1 -> Discrete-Time Integrator1/2
  reset1/1 -> Discrete-Time Integrator/2
  reset/1 -> Discrete-Time Integrator2/2
  u sin(psi)/1 -> Sum1/1
  cos(psi)/1 -> u cos(psi)/1, a w cos(psi)/1
  w/1 -> a w cos(psi)/2, a w sin(psi)/2, Discrete-Time Integrator2/1
  Constant/1 -> a w sin(psi)/1, a w cos(psi)/3
  Discrete-Time Integrator/1 -> x/1
  Sum/1 -> Discrete-Time Integrator/1
  sin(theta)/1 -> a w sin(psi)/3, u sin(psi)/1
  a w cos(psi)/1 -> Sum1/2
  Sum2/1 -> psi/1, sin(theta)/1, cos(psi)/1
  u cos(psi)/1 -> Sum/2
  u/1 -> u sin(psi)/2, u cos(psi)/2
  a w sin(psi)/1 -> Sum/1
  Sum1/1 -> Discrete-Time Integrator1/1
  Discrete-Time Integrator1/1 -> y/1
  Discrete-Time Integrator2/1 -> Sum2/1

== system c6_goto_target/controller1/Subsystem1/Adjust Velocities to Avoid Obstacles/Path Following ==
  SteeringDirection : Inport
  AngularVelocity : Inport  Port=2
  Action Port : ActionPort
  Compute Angular Velocity : MATLAB Function  TreatAsAtomicUnit=on
  Constant : Constant  Value=0
  MaxAngularVelocity : Constant
  Subtract : Sum  Inputs=+-
  dV : Outport  VectorParamsAs1DForOutWhenUnconnected=off
  dW : Outport  Port=2  VectorParamsAs1DForOutWhenUnconnected=off
  wires:
  AngularVelocity/1 -> Subtract/2
  Compute Angular Velocity/1(w) -> Subtract/1
  Subtract/1 -> dW/1
  SteeringDirection/1 -> Compute Angular Velocity/1(steeringDir)
  MaxAngularVelocity/1 -> Compute Angular Velocity/2(wMax)
  Constant/1 -> dV/1

== system c6_goto_target/controller1/Subsystem1/Adjust Velocities to Avoid Obstacles/Recovery ==
  LinearVelocity : Inport
  AngularVelocity : Inport  Port=2
  Action Port : ActionPort
  Constant1 : Constant  Value=recovery_w
  Gain : Gain  Gain=-1
  Subtract : Sum  Inputs=+-
  dV : Outport  VectorParamsAs1DForOutWhenUnconnected=off
  dW : Outport  Port=2  VectorParamsAs1DForOutWhenUnconnected=off
  wires:
  Subtract/1 -> dW/1
  AngularVelocity/1 -> Subtract/2
  Constant1/1 -> Subtract/1
  Gain/1 -> dV/1
  LinearVelocity/1 -> Gain/1

== system c6_goto_target/controller1/Subsystem2/Adjust Velocities to Avoid Obstacles/Path Following ==
  SteeringDirection : Inport
  AngularVelocity : Inport  Port=2
  Action Port : ActionPort
  Compute Angular Velocity : MATLAB Function  TreatAsAtomicUnit=on
  Constant : Constant  Value=0
  MaxAngularVelocity : Constant
  Subtract : Sum  Inputs=+-
  dV : Outport  VectorParamsAs1DForOutWhenUnconnected=off
  dW : Outport  Port=2  VectorParamsAs1DForOutWhenUnconnected=off
  wires:
  Constant/1 -> dV/1
  MaxAngularVelocity/1 -> Compute Angular Velocity/2(wMax)
  SteeringDirection/1 -> Compute Angular Velocity/1(steeringDir)
  Subtract/1 -> dW/1
  Compute Angular Velocity/1(w) -> Subtract/1
  AngularVelocity/1 -> Subtract/2

== system c6_goto_target/controller1/Subsystem2/Adjust Velocities to Avoid Obstacles/Recovery ==
  LinearVelocity : Inport
  AngularVelocity : Inport  Port=2
  Action Port : ActionPort
  Constant1 : Constant  Value=recovery_w
  Gain : Gain  Gain=-1
  Subtract : Sum  Inputs=+-
  dV : Outport  VectorParamsAs1DForOutWhenUnconnected=off
  dW : Outport  Port=2  VectorParamsAs1DForOutWhenUnconnected=off
  wires:
  LinearVelocity/1 -> Gain/1
  Gain/1 -> dV/1
  Constant1/1 -> Subtract/1
  AngularVelocity/1 -> Subtract/2
  Subtract/1 -> dW/1

== system c6_goto_target/controller1/Subsystem3/Adjust Velocities to Avoid Obstacles/Path Following ==
  SteeringDirection : Inport
  AngularVelocity : Inport  Port=2
  Action Port : ActionPort
  Compute Angular Velocity : MATLAB Function  TreatAsAtomicUnit=on
  Constant : Constant  Value=0
  MaxAngularVelocity : Constant
  Subtract : Sum  Inputs=+-
  dV : Outport  VectorParamsAs1DForOutWhenUnconnected=off
  dW : Outport  Port=2  VectorParamsAs1DForOutWhenUnconnected=off
  wires:
  Constant/1 -> dV/1
  MaxAngularVelocity/1 -> Compute Angular Velocity/2(wMax)
  SteeringDirection/1 -> Compute Angular Velocity/1(steeringDir)
  Subtract/1 -> dW/1
  Compute Angular Velocity/1(w) -> Subtract/1
  AngularVelocity/1 -> Subtract/2

== system c6_goto_target/controller1/Subsystem3/Adjust Velocities to Avoid Obstacles/Recovery ==
  LinearVelocity : Inport
  AngularVelocity : Inport  Port=2
  Action Port : ActionPort
  Constant1 : Constant  Value=recovery_w
  Gain : Gain  Gain=-1
  Subtract : Sum  Inputs=+-
  dV : Outport  VectorParamsAs1DForOutWhenUnconnected=off
  dW : Outport  Port=2  VectorParamsAs1DForOutWhenUnconnected=off
  wires:
  LinearVelocity/1 -> Gain/1
  Gain/1 -> dV/1
  Constant1/1 -> Subtract/1
  AngularVelocity/1 -> Subtract/2
  Subtract/1 -> dW/1

== system c6_goto_target/controller1/Subsystem4/Adjust Velocities to Avoid Obstacles/Path Following ==
  SteeringDirection : Inport
  AngularVelocity : Inport  Port=2
  Action Port : ActionPort
  Compute Angular Velocity : MATLAB Function  TreatAsAtomicUnit=on
  Constant : Constant  Value=0
  MaxAngularVelocity : Constant
  Subtract : Sum  Inputs=+-
  dV : Outport  VectorParamsAs1DForOutWhenUnconnected=off
  dW : Outport  Port=2  VectorParamsAs1DForOutWhenUnconnected=off
  wires:
  Constant/1 -> dV/1
  MaxAngularVelocity/1 -> Compute Angular Velocity/2(wMax)
  SteeringDirection/1 -> Compute Angular Velocity/1(steeringDir)
  Subtract/1 -> dW/1
  Compute Angular Velocity/1(w) -> Subtract/1
  AngularVelocity/1 -> Subtract/2

== system c6_goto_target/controller1/Subsystem4/Adjust Velocities to Avoid Obstacles/Recovery ==
  LinearVelocity : Inport
  AngularVelocity : Inport  Port=2
  Action Port : ActionPort
  Constant1 : Constant  Value=recovery_w
  Gain : Gain  Gain=-1
  Subtract : Sum  Inputs=+-
  dV : Outport  VectorParamsAs1DForOutWhenUnconnected=off
  dW : Outport  Port=2  VectorParamsAs1DForOutWhenUnconnected=off
  wires:
  LinearVelocity/1 -> Gain/1
  Gain/1 -> dV/1
  Constant1/1 -> Subtract/1
  AngularVelocity/1 -> Subtract/2
  Subtract/1 -> dW/1

== system c6_goto_target/controller1/Subsystem5/Adjust Velocities to Avoid Obstacles/Path Following ==
  SteeringDirection : Inport
  AngularVelocity : Inport  Port=2
  Action Port : ActionPort
  Compute Angular Velocity : MATLAB Function  TreatAsAtomicUnit=on
  Constant : Constant  Value=0
  MaxAngularVelocity : Constant
  Subtract : Sum  Inputs=+-
  dV : Outport  VectorParamsAs1DForOutWhenUnconnected=off
  dW : Outport  Port=2  VectorParamsAs1DForOutWhenUnconnected=off
  wires:
  Constant/1 -> dV/1
  MaxAngularVelocity/1 -> Compute Angular Velocity/2(wMax)
  SteeringDirection/1 -> Compute Angular Velocity/1(steeringDir)
  Subtract/1 -> dW/1
  Compute Angular Velocity/1(w) -> Subtract/1
  AngularVelocity/1 -> Subtract/2

== system c6_goto_target/controller1/Subsystem5/Adjust Velocities to Avoid Obstacles/Recovery ==
  LinearVelocity : Inport
  AngularVelocity : Inport  Port=2
  Action Port : ActionPort
  Constant1 : Constant  Value=recovery_w
  Gain : Gain  Gain=-1
  Subtract : Sum  Inputs=+-
  dV : Outport  VectorParamsAs1DForOutWhenUnconnected=off
  dW : Outport  Port=2  VectorParamsAs1DForOutWhenUnconnected=off
  wires:
  LinearVelocity/1 -> Gain/1
  Gain/1 -> dV/1
  Constant1/1 -> Subtract/1
  AngularVelocity/1 -> Subtract/2
  Subtract/1 -> dW/1

== system c6_goto_target/controller1/Subsystem6/Adjust Velocities to Avoid Obstacles/Path Following ==
  SteeringDirection : Inport
  AngularVelocity : Inport  Port=2
  Action Port : ActionPort
  Compute Angular Velocity : MATLAB Function  TreatAsAtomicUnit=on
  Constant : Constant  Value=0
  MaxAngularVelocity : Constant
  Subtract : Sum  Inputs=+-
  dV : Outport  VectorParamsAs1DForOutWhenUnconnected=off
  dW : Outport  Port=2  VectorParamsAs1DForOutWhenUnconnected=off
  wires:
  Constant/1 -> dV/1
  MaxAngularVelocity/1 -> Compute Angular Velocity/2(wMax)
  SteeringDirection/1 -> Compute Angular Velocity/1(steeringDir)
  Subtract/1 -> dW/1
  Compute Angular Velocity/1(w) -> Subtract/1
  AngularVelocity/1 -> Subtract/2

== system c6_goto_target/controller1/Subsystem6/Adjust Velocities to Avoid Obstacles/Recovery ==
  LinearVelocity : Inport
  AngularVelocity : Inport  Port=2
  Action Port : ActionPort
  Constant1 : Constant  Value=recovery_w
  Gain : Gain  Gain=-1
  Subtract : Sum  Inputs=+-
  dV : Outport  VectorParamsAs1DForOutWhenUnconnected=off
  dW : Outport  Port=2  VectorParamsAs1DForOutWhenUnconnected=off
  wires:
  LinearVelocity/1 -> Gain/1
  Gain/1 -> dV/1
  Constant1/1 -> Subtract/1
  AngularVelocity/1 -> Subtract/2
  Subtract/1 -> dW/1

== matlab function c6_goto_target/Subsystem/Car Pose Listener2/Subsystem/sensor2vCar4 ==
  data: V output; W output; VW_New input; VW_Msg input
function [V,W] = sensor2vCar(VW_New, VW_Msg)
persistent v0 w0
if isempty(v0)
    v0=0; 
    w0=0;    
end
if VW_New
    v0=VW_Msg.Linear.X;
    w0=VW_Msg.Angular.Z;
end

V=v0;
W=-w0;

== matlab function c6_goto_target/Subsystem/Car Pose Listener1/Subsystem/sensor2vCar ==
  data: x_init output; y_init output; yaw_init output; flag output; poseNew input; poseMsg input
function [x_init,y_init,yaw_init,flag] = sensor2vCar(poseNew, poseMsg)
persistent x0 y0 yaw0 yaw1 x0_init y0_init yaw0_init fStart
if isempty(x0)
    x0=-10; y0=-10; yaw0=0; yaw1=0;   
    x0_init=-10;y0_init=-10;yaw0_init=0;
    fStart=0;
end
if poseNew
    if x0==poseMsg.Pose.Pose.Position.X&&y0==poseMsg.Pose.Pose.Position.Y
        flag=1;
    else
        x0=poseMsg.Pose.Pose.Position.X;
        y0=poseMsg.Pose.Pose.Position.Y;   
        %yaw2=atan2(2*(poseMsg.Pose.Pose.Orientation.Z*poseMsg.Pose.Pose.Orientation.W),1-2*(poseMsg.Pose.Pose.Orientation.Z^2)); 
        eul=quat2eul([poseMsg.Pose.Pose.Orientation.W,poseMsg.Pose.Pose.Orientation.X,poseMsg.Pose.Pose.Orientation.Y,poseMsg.Pose.Pose.Orientation.Z]);
        yaw2=eul(1);
        %对前后角度差使用积分，恢复yaw的连续性
        yaw0=yaw0+angdiff(yaw1,yaw2);
        yaw1=yaw2;
        flag=0;        
        x0_init=x0;
        y0_init=y0;
        yaw0_init=yaw0;
        fStart=1;
    end 
else
    if fStart
        flag=1;
    else
        flag=0;
    end
end

x_init=x0_init;y_init=y0_init;yaw_init=yaw0_init;

== matlab function c6_goto_target/Subsystem/Car Pose Listener1/Subsystem/sensor2vCar4 ==
  data: V output; W output; VW_New input; VW_Msg input
function [V,W] = sensor2vCar(VW_New, VW_Msg)
persistent v0 w0
if isempty(v0)
    v0=0; 
    w0=0;    
end
if VW_New
    v0=VW_Msg.Linear.X;
    w0=VW_Msg.Angular.Z;
end

V=v0;
W=-w0;

== matlab function c6_goto_target/Subsystem/Car Pose Listener/Subsystem/sensor2vCar ==
  data: x_init output; y_init output; yaw_init output; flag output; poseNew input; poseMsg input
function [x_init,y_init,yaw_init,flag] = sensor2vCar(poseNew, poseMsg)
persistent x0 y0 yaw0 yaw1 x0_init y0_init yaw0_init fStart
if isempty(x0)
    x0=-10; y0=-10; yaw0=0; yaw1=0;   
    x0_init=-10;y0_init=-10;yaw0_init=0;
    fStart=0;
end
if poseNew
    if x0==poseMsg.Pose.Pose.Position.X&&y0==poseMsg.Pose.Pose.Position.Y
        flag=1;
    else
        x0=poseMsg.Pose.Pose.Position.X;
        y0=poseMsg.Pose.Pose.Position.Y;   
        %yaw2=atan2(2*(poseMsg.Pose.Pose.Orientation.Z*poseMsg.Pose.Pose.Orientation.W),1-2*(poseMsg.Pose.Pose.Orientation.Z^2)); 
        eul=quat2eul([poseMsg.Pose.Pose.Orientation.W,poseMsg.Pose.Pose.Orientation.X,poseMsg.Pose.Pose.Orientation.Y,poseMsg.Pose.Pose.Orientation.Z]);
        yaw2=eul(1);
        %对前后角度差使用积分，恢复yaw的连续性
        yaw0=yaw0+angdiff(yaw1,yaw2);
        yaw1=yaw2;
        flag=0;        
        x0_init=x0;
        y0_init=y0;
        yaw0_init=yaw0;
        fStart=1;
    end 
else
    if fStart
        flag=1;
    else
        flag=0;
    end
end

x_init=x0_init;y_init=y0_init;yaw_init=yaw0_init;

== matlab function c6_goto_target/Subsystem/Car Pose Listener/Subsystem/sensor2vCar4 ==
  data: V output; W output; VW_New input; VW_Msg input
function [V,W] = sensor2vCar(VW_New, VW_Msg)
persistent v0 w0
if isempty(v0)
    v0=0; 
    w0=0;    
end
if VW_New
    v0=VW_Msg.Linear.X;
    w0=VW_Msg.Angular.Z;
end

V=v0;
W=-w0;

== matlab function c6_goto_target/controller1/Subsystem1/Adjust Velocities to Avoid Obstacles/Path Following/Compute Angular Velocity ==
  data: steeringDir input; w output; wMax input
function w = exampleHelperComputeAngularVelocity(steeringDir, wMax)
%EXAMPLEHELPERCOMPUTEANGULARVELOCITY Compute angular velocity
%   W = exampleHelperComputeAngularVelocity(STEERINGDIR)
%   returns the angular velocity W for a differential drive robot in radians
%   per second for a given steering direction STEERINGDIR in the robot's
%   coordinate frame in radians.
%
%   W = exampleHelperComputeAngularVelocity(STEERINGDIR, WMAX)
%   returns the angular velocity W for a differential drive robot in radians
%   per second for a given steering direction STEERINGDIR in the robot's
%   coordinate frame in radians and maximum angular velocity WMAX in
%   radians per second. The output angular velocity is saturated based on
%   the WMAX.
%
%   Example:
%       
%       w = exampleHelperComputeAngularVelocity(0.2, 1);

% Copyright 2015 The MathWorks, Inc.

%#codegen
%#ok<*EMCA>

% Allow variable input arguments
if nargin == 1   
    wMax = inf;
end

validateattributes(steeringDir, {'double'},{'real'},...
    'exampleHelperComputeAngularVelocity', 'STEERINGDIR', 1);
validateattributes(wMax, {'double'},{'real', 'positive'},...
    'exampleHelperComputeAngularVelocity', 'WMAX', 2);

% Computing in robot's coordinate frame
curPose = [0 0 0];

% The following computation is similar to robotics.PurePursuit
lookaheadPoint = [cos(steeringDir), sin(steeringDir)];
slope = atan2((lookaheadPoint(2) - curPose(2)), ...
    (lookaheadPoint(1) - curPose(1)));
alpha = angdiff(curPose(3), slope);

% Angular velocity command for a differential drive robot is
% equal to the desired curvature to be followed by the robot.

w = (2*sin(alpha));

% Pick a constant rotation when robot is facing in the opposite
% direction of the path
if abs(abs(alpha) - pi) < 1e-12
    w = sign(w)*1;
end

if abs(w) > wMax
    w = sign(w)*wMax;
end

end

== matlab function c6_goto_target/controller1/Subsystem1/Compute Velocity and Heading for Path following/ Extract Goal ==
  data: Waypoints input; Goal output
function Goal = extractGoal(Waypoints)
%#codegen
b = isnan(Waypoints);
[rows,~] = find(b);
ridx = setdiff(1:size(Waypoints,1), sort(rows));
Goal = [Waypoints(ridx(end), 1) Waypoints(ridx(end), 2)];

== matlab function c6_goto_target/controller1/MATLAB Function ==
  data: t1 output; t2 output; t3 output; t4 output; t5 output; t6 output; a input; wp1 input
function [t1,t2,t3,t4,t5,t6] = go2target(a,wp1)

%取每位值
 
if a>900000||a<100000
    a=123456;
end
% 
% A=0.3;
% C=1.7;
% B=(A+C)/2;
% 
% wp1=[A,A; B,A;  C,A;
%  C,B;
% C,C; B,C; A,C;
% A,B;A,A]; 

a1=fix(a/100000);
a2=fix(mod(a,100000)/10000);
a3=fix(mod(a,10000)/1000);
a4=fix(mod(a,1000)/100);
a5=fix(mod(a,100)/10);
a6=mod(a,10);

 
 
 
t1=wp1(a1,:);
t2=wp1(a2,:);
t3=wp1(a3,:);
t4=wp1(a4,:);
t5=wp1(a5,:);
t6=wp1(a6,:);

== matlab function c6_goto_target/controller1/Subsystem2/Adjust Velocities to Avoid Obstacles/Path Following/Compute Angular Velocity ==
  data: steeringDir input; w output; wMax input
function w = exampleHelperComputeAngularVelocity(steeringDir, wMax)
%EXAMPLEHELPERCOMPUTEANGULARVELOCITY Compute angular velocity
%   W = exampleHelperComputeAngularVelocity(STEERINGDIR)
%   returns the angular velocity W for a differential drive robot in radians
%   per second for a given steering direction STEERINGDIR in the robot's
%   coordinate frame in radians.
%
%   W = exampleHelperComputeAngularVelocity(STEERINGDIR, WMAX)
%   returns the angular velocity W for a differential drive robot in radians
%   per second for a given steering direction STEERINGDIR in the robot's
%   coordinate frame in radians and maximum angular velocity WMAX in
%   radians per second. The output angular velocity is saturated based on
%   the WMAX.
%
%   Example:
%       
%       w = exampleHelperComputeAngularVelocity(0.2, 1);

% Copyright 2015 The MathWorks, Inc.

%#codegen
%#ok<*EMCA>

% Allow variable input arguments
if nargin == 1   
    wMax = inf;
end

validateattributes(steeringDir, {'double'},{'real'},...
    'exampleHelperComputeAngularVelocity', 'STEERINGDIR', 1);
validateattributes(wMax, {'double'},{'real', 'positive'},...
    'exampleHelperComputeAngularVelocity', 'WMAX', 2);

% Computing in robot's coordinate frame
curPose = [0 0 0];

% The following computation is similar to robotics.PurePursuit
lookaheadPoint = [cos(steeringDir), sin(steeringDir)];
slope = atan2((lookaheadPoint(2) - curPose(2)), ...
    (lookaheadPoint(1) - curPose(1)));
alpha = angdiff(curPose(3), slope);

% Angular velocity command for a differential drive robot is
% equal to the desired curvature to be followed by the robot.

w = (2*sin(alpha));

% Pick a constant rotation when robot is facing in the opposite
% direction of the path
if abs(abs(alpha) - pi) < 1e-12
    w = sign(w)*1;
end

if abs(w) > wMax
    w = sign(w)*wMax;
end

end
